simulink model "two_vehicle_pub_sub_scenario"  (R2024a)
settings: Solver=VariableStepAuto  StartTime=0.0  StopTime=inf  FixedStep=0.1  RelTol=1e-3
undefined symbols (not defined in the file): DiscIntNeverNeededParam, x, y
libraries: ros2lib x12
settings Model: Creator=ruby  LastModifiedBy=ruby

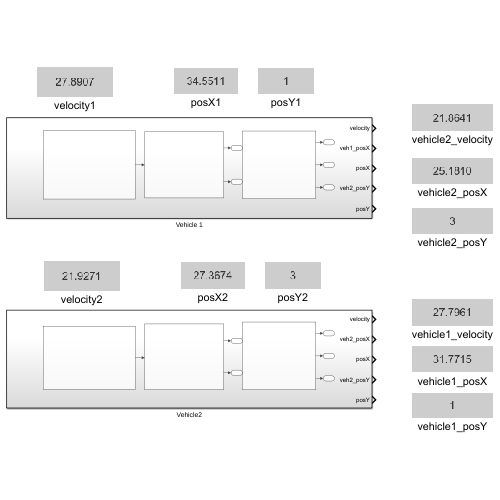
[thumbnail: Simulink's stored preview of the top-level diagram]
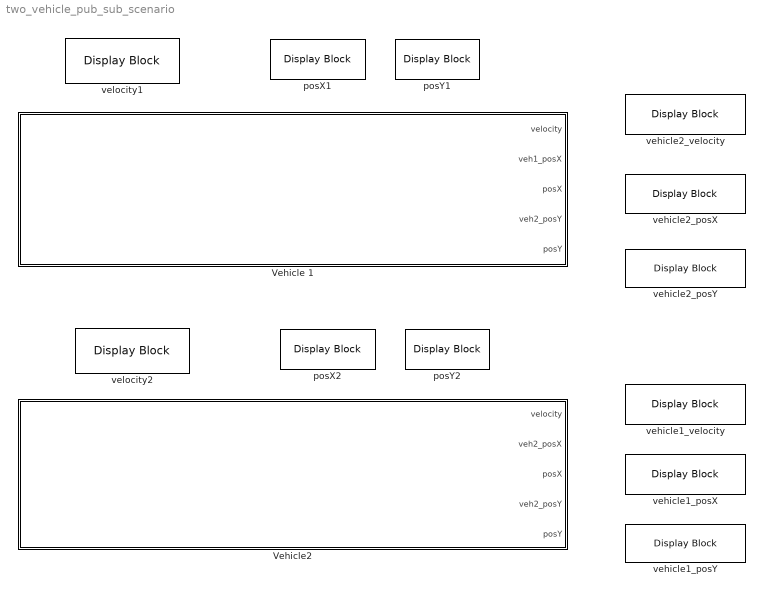
== system two_vehicle_pub_sub_scenario ==
  Vehicle 1 : Subsystem
  Vehicle2 : Subsystem
  posX1 : DisplayBlock  LabelPosition=Hide  Transparency=1
  posX2 : DisplayBlock  LabelPosition=Hide  Transparency=1
  posY1 : DisplayBlock  LabelPosition=Hide  Transparency=1
  posY2 : DisplayBlock  LabelPosition=Hide  Transparency=1
  vehicle1_posX : DisplayBlock  LabelPosition=Hide  Transparency=1
  vehicle1_posY : DisplayBlock  LabelPosition=Hide  Transparency=1
  vehicle1_velocity : DisplayBlock  LabelPosition=Hide  Transparency=1
  vehicle2_posX : DisplayBlock  LabelPosition=Hide  Transparency=1
  vehicle2_posY : DisplayBlock  LabelPosition=Hide  Transparency=1
  vehicle2_velocity : DisplayBlock  LabelPosition=Hide  Transparency=1
  velocity1 : DisplayBlock  LabelPosition=Hide  Transparency=1
  velocity2 : DisplayBlock  LabelPosition=Hide  Transparency=1

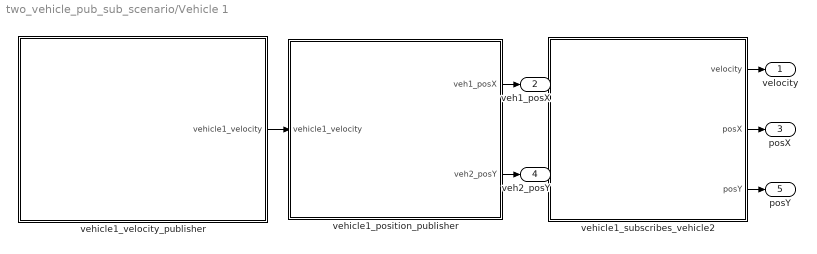
== system two_vehicle_pub_sub_scenario/Vehicle 1 ==
  vehicle1_position_publisher : Subsystem
  vehicle1_subscribes_vehicle2 : Subsystem
  vehicle1_velocity_publisher : Subsystem
  velocity : Outport
  veh1_posX : Outport  Port=2
  posX : Outport  Port=3
  veh2_posY : Outport  Port=4
  posY : Outport  Port=5
  wires:
  vehicle1_velocity_publisher/1(vehicle1_velocity) -> vehicle1_position_publisher/1(vehicle1_velocity)
  vehicle1_position_publisher/1(veh1_posX) -> veh1_posX/1
  vehicle1_position_publisher/2(veh2_posY) -> veh2_posY/1
  vehicle1_subscribes_vehicle2/1(velocity) -> velocity/1
  vehicle1_subscribes_vehicle2/2(posX) -> posX/1
  vehicle1_subscribes_vehicle2/3(posY) -> posY/1

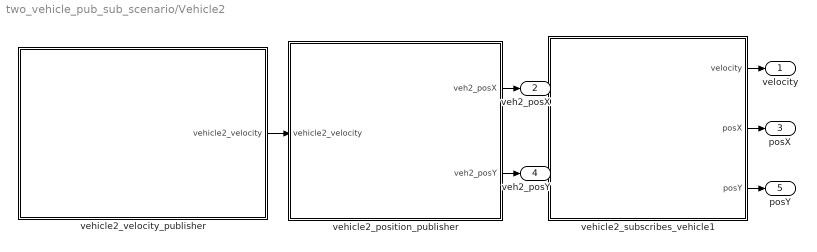
== system two_vehicle_pub_sub_scenario/Vehicle2 ==
  vehicle2_position_publisher : Subsystem
  vehicle2_subscribes_vehicle1 : Subsystem
  vehicle2_velocity_publisher : Subsystem
  velocity : Outport
  veh2_posX : Outport  Port=2
  posX : Outport  Port=3
  veh2_posY : Outport  Port=4
  posY : Outport  Port=5
  wires:
  vehicle2_velocity_publisher/1(vehicle2_velocity) -> vehicle2_position_publisher/1(vehicle2_velocity)
  vehicle2_subscribes_vehicle1/3(posY) -> posY/1
  vehicle2_position_publisher/2(veh2_posY) -> veh2_posY/1
  vehicle2_subscribes_vehicle1/1(velocity) -> velocity/1
  vehicle2_position_publisher/1(veh2_posX) -> veh2_posX/1
  vehicle2_subscribes_vehicle1/2(posX) -> posX/1

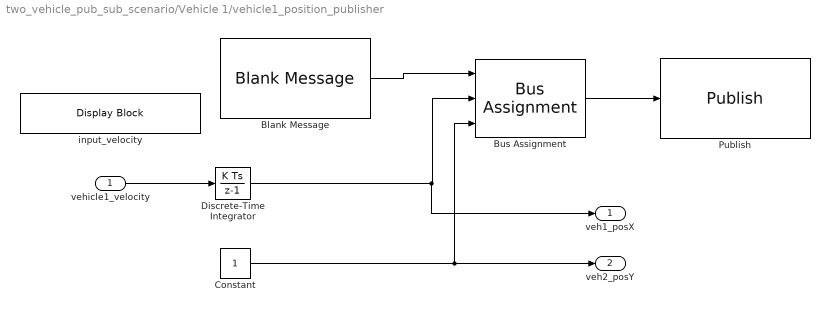
== system two_vehicle_pub_sub_scenario/Vehicle 1/vehicle1_position_publisher ==
  vehicle1_velocity : Inport
  Blank Message : ros2lib/Blank Message  messageClass=Message  entityType=geometry_msgs/Point  messageType=geometry_msgs/Point  SampleTime=inf
  Bus Assignment : BusAssignment  AssignedSignals=x,y
  Constant : Constant
  Discrete-Time Integrator : DiscreteIntegrator  SampleTime=0.1  ICPrevOutput=DiscIntNeverNeededParam  ICPrevScaledInput=DiscIntNeverNeededParam
  Publish : ros2lib/Publish  topicSource=Specify your own  topic=/vehicle1/position  messageType=geometry_msgs/Point  QOSHistory=Keep last  QOSDepth=1  QOSReliability=Reliable  QOSDurability=Volatile  QOSDeadline=Inf  QOSLifespan=Inf  QOSLiveliness=Automatic  QOSLeaseDuration=Inf  QOSAvoidROSNamespaceConventions=off
  input_velocity : DisplayBlock  LabelPosition=Hide  Transparency=1
  veh1_posX : Outport
  veh2_posY : Outport  Port=2
  wires:
  Discrete-Time Integrator/1 -> veh1_posX/1, Bus Assignment/2
  Bus Assignment/1 -> Publish/1
  Blank Message/1 -> Bus Assignment/1
  Constant/1 -> veh2_posY/1, Bus Assignment/3
  vehicle1_velocity/1 -> Discrete-Time Integrator/1

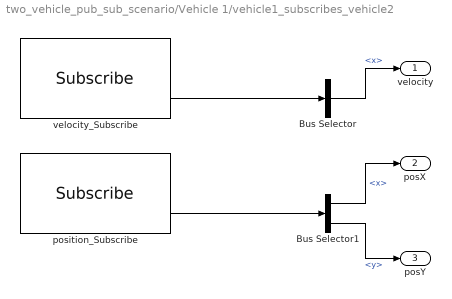
== system two_vehicle_pub_sub_scenario/Vehicle 1/vehicle1_subscribes_vehicle2 ==
  Bus Selector : BusSelector  OutputSignals=linear.x
  Bus Selector1 : BusSelector  OutputSignals=x,y
  position_Subscribe : ros2lib/Subscribe  topicSource=Specify your own  topic=/vehicle2/position  messageType=geometry_msgs/Point  sampleTime=0.1  QOSHistory=Keep last  QOSDepth=1  QOSReliability=Reliable  QOSDurability=Volatile  QOSDeadline=Inf  QOSLifespan=Inf  QOSLiveliness=Automatic  QOSLeaseDuration=Inf  QOSAvoidROSNamespaceConventions=off
  velocity_Subscribe : ros2lib/Subscribe  topicSource=Specify your own  topic=/vehicle2/velocity  messageType=geometry_msgs/Twist  sampleTime=0.1  QOSHistory=Keep last  QOSDepth=1  QOSReliability=Reliable  QOSDurability=Volatile  QOSDeadline=Inf  QOSLifespan=Inf  QOSLiveliness=Automatic  QOSLeaseDuration=Inf  QOSAvoidROSNamespaceConventions=off
  velocity : Outport
  posX : Outport  Port=2
  posY : Outport  Port=3
  wires:
  position_Subscribe/2 -> Bus Selector1/1
  Bus Selector/1 -> velocity/1  "<x>"
  velocity_Subscribe/2 -> Bus Selector/1
  Bus Selector1/1 -> posX/1  "<x>"
  Bus Selector1/2 -> posY/1  "<y>"

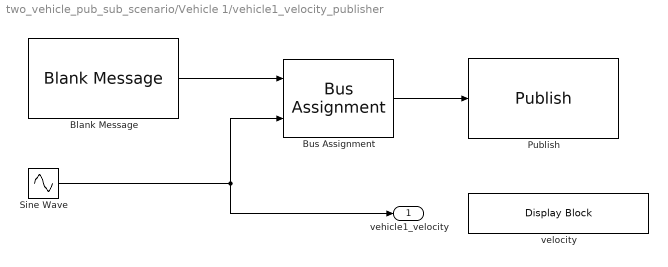
== system two_vehicle_pub_sub_scenario/Vehicle 1/vehicle1_velocity_publisher ==
  Blank Message : ros2lib/Blank Message  messageClass=Message  entityType=geometry_msgs/Twist  messageType=geometry_msgs/Twist  SampleTime=inf
  Bus Assignment : BusAssignment  AssignedSignals=linear.x
  Publish : ros2lib/Publish  topicSource=Specify your own  topic=/vehicle1/velocity  messageType=geometry_msgs/Twist  QOSHistory=Keep last  QOSDepth=1  QOSReliability=Reliable  QOSDurability=Volatile  QOSDeadline=Inf  QOSLifespan=Inf  QOSLiveliness=Automatic  QOSLeaseDuration=Inf  QOSAvoidROSNamespaceConventions=off
  Sine Wave : Sin  Amplitude=3  Bias=25  SampleTime=0.1
  velocity : DisplayBlock  LabelPosition=Hide  Transparency=1
  vehicle1_velocity : Outport
  wires:
  Sine Wave/1 -> vehicle1_velocity/1, Bus Assignment/2
  Bus Assignment/1 -> Publish/1
  Blank Message/1 -> Bus Assignment/1

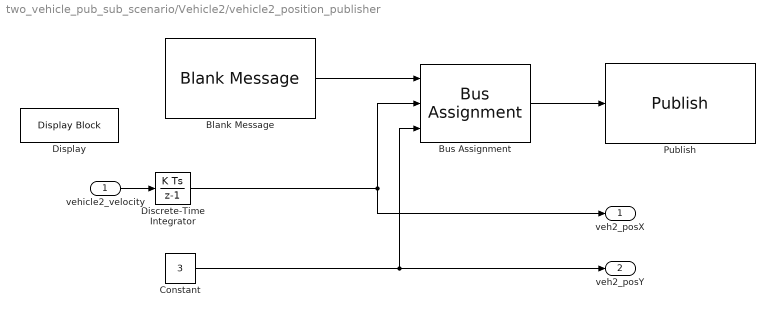
== system two_vehicle_pub_sub_scenario/Vehicle2/vehicle2_position_publisher ==
  vehicle2_velocity : Inport
  Blank Message : ros2lib/Blank Message  messageClass=Message  entityType=geometry_msgs/Point  messageType=geometry_msgs/Point  SampleTime=inf
  Bus Assignment : BusAssignment  AssignedSignals=x,y
  Constant : Constant  Value=3
  Discrete-Time Integrator : DiscreteIntegrator  SampleTime=-1  ICPrevOutput=DiscIntNeverNeededParam  ICPrevScaledInput=DiscIntNeverNeededParam
  Display : DisplayBlock  LabelPosition=Hide  Transparency=1
  Publish : ros2lib/Publish  topicSource=Specify your own  topic=/vehicle2/position  messageType=geometry_msgs/Point  QOSHistory=Keep last  QOSDepth=1  QOSReliability=Reliable  QOSDurability=Volatile  QOSDeadline=Inf  QOSLifespan=Inf  QOSLiveliness=Automatic  QOSLeaseDuration=Inf  QOSAvoidROSNamespaceConventions=off
  veh2_posX : Outport
  veh2_posY : Outport  Port=2
  wires:
  Discrete-Time Integrator/1 -> veh2_posX/1, Bus Assignment/2
  Bus Assignment/1 -> Publish/1
  Blank Message/1 -> Bus Assignment/1
  Constant/1 -> veh2_posY/1, Bus Assignment/3
  vehicle2_velocity/1 -> Discrete-Time Integrator/1

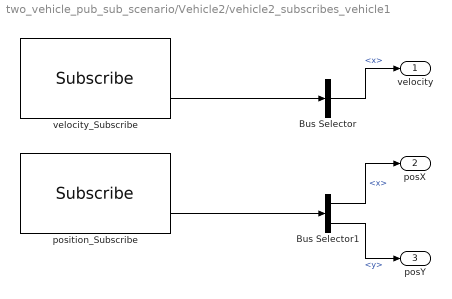
== system two_vehicle_pub_sub_scenario/Vehicle2/vehicle2_subscribes_vehicle1 ==
  Bus Selector : BusSelector  OutputSignals=linear.x
  Bus Selector1 : BusSelector  OutputSignals=x,y
  position_Subscribe : ros2lib/Subscribe  topicSource=Specify your own  topic=/vehicle1/position  messageType=geometry_msgs/Point  sampleTime=0.1  QOSHistory=Keep last  QOSDepth=1  QOSReliability=Reliable  QOSDurability=Volatile  QOSDeadline=Inf  QOSLifespan=Inf  QOSLiveliness=Automatic  QOSLeaseDuration=Inf  QOSAvoidROSNamespaceConventions=off
  velocity_Subscribe : ros2lib/Subscribe  topicSource=Specify your own  topic=/vehicle1/velocity  messageType=geometry_msgs/Twist  sampleTime=0.1  QOSHistory=Keep last  QOSDepth=1  QOSReliability=Reliable  QOSDurability=Volatile  QOSDeadline=Inf  QOSLifespan=Inf  QOSLiveliness=Automatic  QOSLeaseDuration=Inf  QOSAvoidROSNamespaceConventions=off
  velocity : Outport
  posX : Outport  Port=2
  posY : Outport  Port=3
  wires:
  position_Subscribe/2 -> Bus Selector1/1
  Bus Selector/1 -> velocity/1  "<x>"
  velocity_Subscribe/2 -> Bus Selector/1
  Bus Selector1/1 -> posX/1  "<x>"
  Bus Selector1/2 -> posY/1  "<y>"

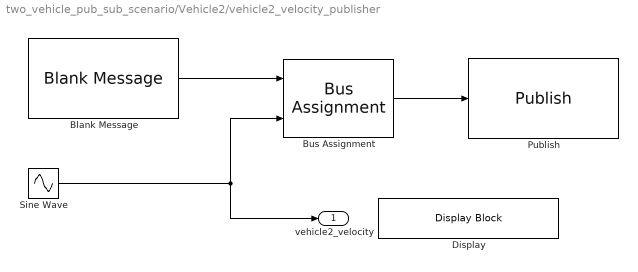
== system two_vehicle_pub_sub_scenario/Vehicle2/vehicle2_velocity_publisher ==
  Blank Message : ros2lib/Blank Message  messageClass=Message  entityType=geometry_msgs/Twist  messageType=geometry_msgs/Twist  SampleTime=inf
  Bus Assignment : BusAssignment  AssignedSignals=linear.x
  Display : DisplayBlock  LabelPosition=Hide  Transparency=1
  Publish : ros2lib/Publish  topicSource=Specify your own  topic=/vehicle2/velocity  messageType=geometry_msgs/Twist  QOSHistory=Keep last  QOSDepth=1  QOSReliability=Reliable  QOSDurability=Volatile  QOSDeadline=Inf  QOSLifespan=Inf  QOSLiveliness=Automatic  QOSLeaseDuration=Inf  QOSAvoidROSNamespaceConventions=off
  Sine Wave : Sin  Amplitude=2  Bias=20  SampleTime=0.1
  vehicle2_velocity : Outport
  wires:
  Sine Wave/1 -> Bus Assignment/2, vehicle2_velocity/1
  Bus Assignment/1 -> Publish/1
  Blank Message/1 -> Bus Assignment/1
